simulink model "DecoderStepCLEARlModel"  (R2016b)
settings: Solver=FixedStepAuto  StartTime=0.0  StopTime=inf  FixedStep=sCoreParams.core.stepPeriod*50  RelTol=1e-3  SampleTimeConstraint=STIndependent  EnableMultiTasking=on
undefined symbols (not defined in the file): neuralModelParams
settings Model: Creator=anish  LastModifiedBy=rzelmann
settings SolverCC: EnableConcurrentExecution=on
settings DataIOCC: SaveFormat=StructureWithTime  SignalLoggingSaveFormat=ModelDataLogs  SaveOutput=off  SignalLogging=off  DSMLogging=off  SaveTime=off
settings OptimizationCC: BlockReduction=off  ConditionallyExecuteInputs=off  DefaultParameterBehavior=Inlined  OptimizeBlockIOStorage=off  BufferReuse=off  GlobalBufferReuse=off  ExpressionFolding=off  LocalBlockOutputs=off  LifeSpan=inf
settings DebuggingCC: SignalRangeChecking=error  SaveWithParameterizedLinksMsg=none  AllowSymbolicDim=off  ModelReferenceSymbolNameMessage=none  StateNameClashWarn=warning  SFUnexpectedBacktrackingDiag=warning  SFNoUnconditionalDefaultTransitionDiag=warning  SFExecutionAtInitializationDiag=none
settings HardwareCC: ProdBitPerPointer=32  ProdBitPerSizeT=32  ProdBitPerPtrDiffT=32  ProdLargestAtomicFloat=None  ProdWordSize=32  ProdLongLongMode=on  ProdHWDeviceType=Generic->32-bit x86 compatible  TargetBitPerPointer=64  TargetLargestAtomicFloat=Float  TargetLongLongMode=on  TargetIntDivRoundTo=Zero  TargetEndianess=LittleEndian  TargetWordSize=64  TargetHWDeviceType=Intel->x86-64 (Windows64)
settings ModelReferenceCC: UpdateModelReferenceTargets=Force  ModelReferenceNumInstancesAllowed=Single  ModelReferencePassRootInputsByReference=off
settings RTWCC: SystemTargetFile=slrt.tlc  TemplateMakefile=slrt_default_tmf  Description=Simulink Real-Time  BuildConfiguration=Faster Runs  RTWCompilerOptimization=on
settings ConfigComp: CovMetricSettings=dw  CovHtmlReporting=on  CovSaveCumulativeToWorkspaceVar=on  CovSaveSingleToWorkspaceVar=on  CovExternalEMLEnable=off  CovSFcnEnable=off

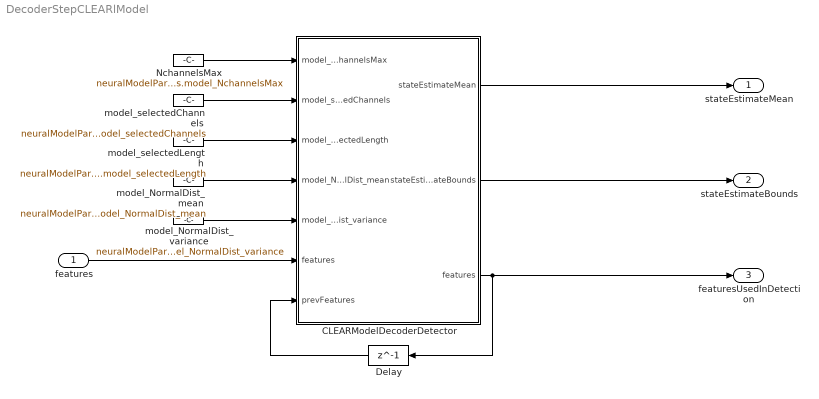
== system DecoderStepCLEARlModel ==
  features : Inport  PortDimensions=[neuralModelParams.nDataPoints neuralModelParams.nFeatures]
  CLEARModelDecoderDetector : MATLAB Function  TreatAsAtomicUnit=on
  Delay : Delay  DelayLength=1
  NchannelsMax : Constant  Value=neuralModelParams.model_NchannelsMax
  model_NormalDist_mean : Constant  Value=neuralModelParams.model_NormalDist_mean
  model_NormalDist_variance : Constant  Value=neuralModelParams.model_NormalDist_variance
  model_selectedChannels : Constant  Value=neuralModelParams.model_selectedChannels
  model_selectedLength : Constant  Value=neuralModelParams.model_selectedLength
  stateEstimateMean : Outport  InitialOutput=-500
  stateEstimateBounds : Outport  Port=2  InitialOutput=[-500 -500]
  featuresUsedInDetection : Outport  Port=3
  wires:
  CLEARModelDecoderDetector/1(stateEstimateMean) -> stateEstimateMean/1
  Delay/1 -> CLEARModelDecoderDetector/7(prevFeatures)
  model_selectedChannels/1 -> CLEARModelDecoderDetector/2(model_selectedChannels)
  model_NormalDist_mean/1 -> CLEARModelDecoderDetector/4(model_NormalDist_mean)
  model_NormalDist_variance/1 -> CLEARModelDecoderDetector/5(model_NormalDist_variance)
  features/1 -> CLEARModelDecoderDetector/6("features ")
  CLEARModelDecoderDetector/3(features) -> featuresUsedInDetection/1, Delay/1
  CLEARModelDecoderDetector/2(stateEstimateBounds) -> stateEstimateBounds/1
  NchannelsMax/1 -> CLEARModelDecoderDetector/1(model_NchannelsMax)
  model_selectedLength/1 -> CLEARModelDecoderDetector/3(model_selectedLength)

== matlab function DecoderStepCLEARlModel/CLEARModelDecoderDetector ==
  data: stateEstimateMean output; stateEstimateBounds output size=[1 2]; model_NchannelsMax input; model_selectedChannels input; model_selectedLength input; model_NormalDist_mean input; model_NormalDist_variance input; features output; features input; prevFeatures input
function [stateEstimateMean, stateEstimateBounds, features] = CLEARModelDecoderDetector( model_NchannelsMax, model_selectedChannels,model_selectedLength, model_NormalDist_mean, model_NormalDist_variance, features, prevFeatures)
%#codegen

stateEstimateMean =0;
% features is transpose to accomodate model input - RIZ: could be removed in the future once model is stable and we can swap direction in it!
[output] = nz_predict_CLoSES(model_NchannelsMax, model_selectedChannels, model_selectedLength, model_NormalDist_mean, model_NormalDist_variance, features');
stateEstimateMean = output; %Estimate.Mean;
stateEstimateBounds = [output output]; %Estimate.Bound;
